simulink model "Motor_controller"  (R2014a)
settings: Solver=ode45  StartTime=0.0  StopTime=10.0  RelTol=1e-3
model workspace: external: MAT-File WaveSculptor_200.mat (data not in the file)
undefined symbols (not defined in the file or in its folder): Motor_Cutout_Temperature, Motor_Ramp_Temperature, Sine_Current_Limit
settings Model: Creator=abk  LastModifiedBy=Nathan
settings DataIOCC: LimitDataPoints=off

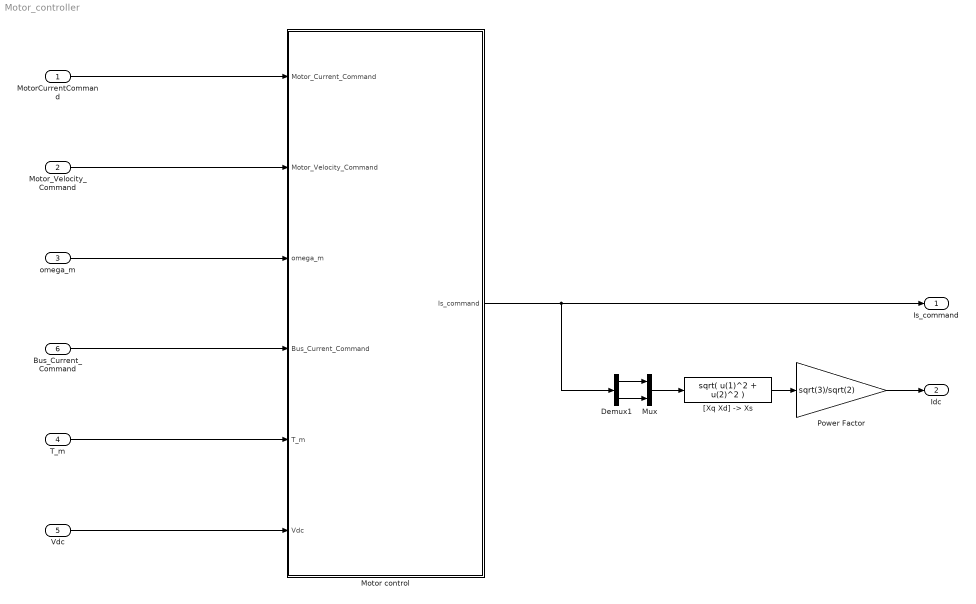
== system Motor_controller ==
  MotorCurrentCommand : Inport
  Motor_Velocity_Command : Inport  Port=2
  omega_m : Inport  Port=3
  T_m : Inport  Port=4
  Vdc : Inport  Port=5
  Bus_Current_Command : Inport  Port=6
  Demux1 : Demux  Outputs=2
  Motor control : Subsystem
  Mux : Mux  Inputs=2
  Power Factor : Gain  Gain=sqrt(3)/sqrt(2)
  "[Xq Xd] -> Xs" : Fcn  Expr=sqrt( u(1)^2 + u(2)^2 )
  Is_command : Outport  OutDataTypeStr=Bus: Is_bus  BusOutputAsStruct=on
  Idc : Outport  Port=2
  wires:
  MotorCurrentCommand/1 -> Motor control/1(Motor_Current_Command)
  Motor_Velocity_Command/1 -> Motor control/2(Motor_Velocity_Command)
  omega_m/1 -> Motor control/3(omega_m)
  Bus_Current_Command/1 -> Motor control/4(Bus_Current_Command)
  T_m/1 -> Motor control/5(T_m)
  Vdc/1 -> Motor control/6(Vdc)
  Power Factor/1 -> Idc/1
  Motor control/1(Is_command) -> Demux1/1, Is_command/1
  Demux1/1 -> Mux/1
  Demux1/2 -> Mux/2
  Mux/1 -> "[Xq Xd] -> Xs"/1
  "[Xq Xd] -> Xs"/1 -> Power Factor/1

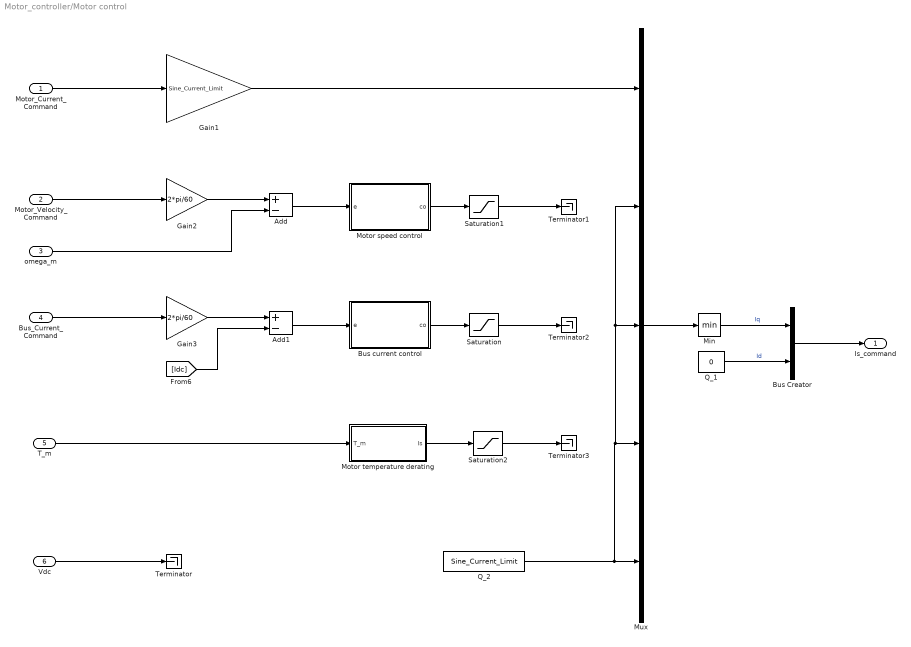
== system Motor_controller/Motor control ==
  Motor_Current_Command : Inport
  Motor_Velocity_Command : Inport  Port=2
  omega_m : Inport  Port=3
  Bus_Current_Command : Inport  Port=4
  T_m : Inport  Port=5
  Vdc : Inport  Port=6
  Add : Sum  Inputs=+-
  Add1 : Sum  Inputs=+-
  Bus Creator : BusCreator  Inputs=2
  Bus current control : Subsystem
  Gain1 : Gain  Gain=Sine_Current_Limit
  Gain2 : Gain  Gain=2*pi/60
  Gain3 : Gain  Gain=2*pi/60
  Min : MinMax
  Motor speed control : Subsystem
  "Motor temperature derating " : Subsystem
  Mux : Mux  Inputs=5
  Q_1 : Constant  Value=0
  Q_2 : Constant  Value=Sine_Current_Limit
  Saturation : Saturate  UpperLimit=Sine_Current_Limit  LowerLimit=-Sine_Current_Limit
  Saturation1 : Saturate  UpperLimit=Sine_Current_Limit  LowerLimit=-Sine_Current_Limit
  Saturation2 : Saturate  UpperLimit=Sine_Current_Limit  LowerLimit=-Sine_Current_Limit
  Terminator{,1..3} (4 alike) : Terminator
  Is_command : Outport
  wires:
  Motor_Velocity_Command/1 -> Gain2/1
  Vdc/1 -> Terminator/1
  Gain2/1 -> Add/1
  Motor speed control/1(co) -> Saturation1/1
  Bus current control/1(co) -> Saturation/1
  Add/1 -> Motor speed control/1("e ")
  omega_m/1 -> Add/2
  Motor_Current_Command/1 -> Gain1/1
  T_m/1 -> "Motor temperature derating "/1(T_m)
  "Motor temperature derating "/1(Is) -> Saturation2/1
  Bus_Current_Command/1 -> Gain3/1
  Gain3/1 -> Add1/1
  [Idc] -> Add1/2
  Add1/1 -> Bus current control/1("e ")
  Min/1 -> Bus Creator/1  "Iq"
  Q_1/1 -> Bus Creator/2  "Id"
  Bus Creator/1 -> Is_command/1
  Gain1/1 -> Mux/1
  Mux/1 -> Min/1
  Saturation2/1 -> Terminator3/1
  Saturation/1 -> Terminator2/1
  Saturation1/1 -> Terminator1/1
  Q_2/1 -> Mux/2, Mux/3, Mux/4, Mux/5

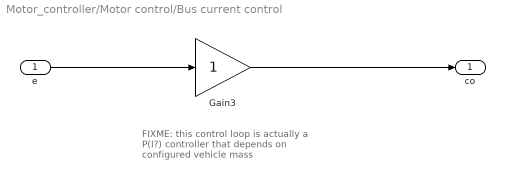
== system Motor_controller/Motor control/Bus current control ==
  note: FIXME: this control loop is actually a P(I?) controller that depends on configured vehicle mass
  "e " : Inport
  Gain3 : Gain
  co : Outport
  wires:
  "e "/1 -> Gain3/1
  Gain3/1 -> co/1

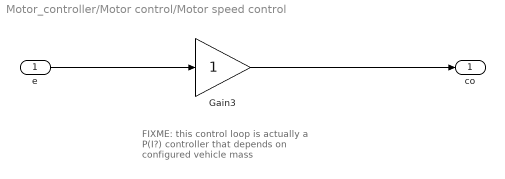
== system Motor_controller/Motor control/Motor speed control ==
  note: FIXME: this control loop is actually a P(I?) controller that depends on configured vehicle mass
  "e " : Inport
  Gain3 : Gain
  co : Outport
  wires:
  "e "/1 -> Gain3/1
  Gain3/1 -> co/1

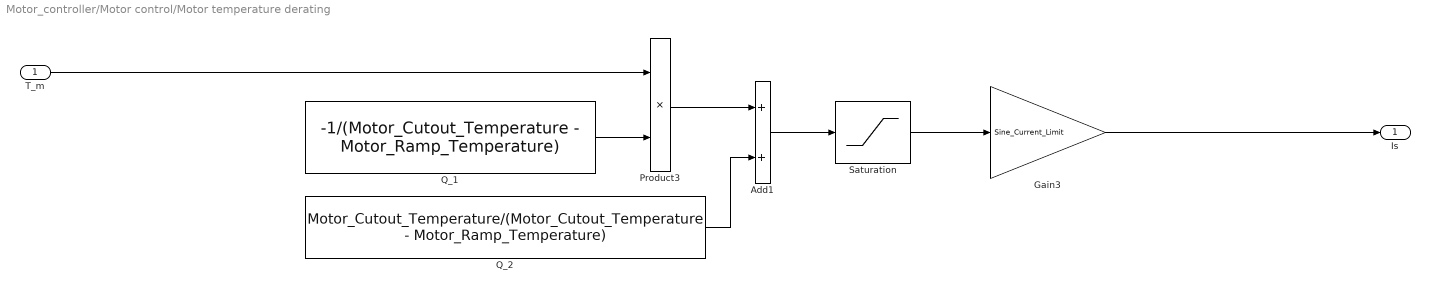
== system Motor_controller/Motor control/Motor temperature derating  ==
  T_m : Inport
  Add1 : Sum
  Gain3 : Gain  Gain=Sine_Current_Limit
  Product3 : Product
  Q_1 : Constant  Value=-1/(Motor_Cutout_Temperature - Motor_Ramp_Temperature)
  Q_2 : Constant  Value=Motor_Cutout_Temperature/(Motor_Cutout_Temperature - Motor_Ramp_Temperature)
  Saturation : Saturate  UpperLimit=1  LowerLimit=0
  Is : Outport
  wires:
  Q_1/1 -> Product3/2
  T_m/1 -> Product3/1
  Q_2/1 -> Add1/2
  Gain3/1 -> Is/1
  Add1/1 -> Saturation/1
  Product3/1 -> Add1/1
  Saturation/1 -> Gain3/1
